simulink model "iiwa_model_tests"  (R2020b)
settings: Solver=VariableStepAuto  StartTime=0.0  StopTime=10.0  RelTol=1e-3
values from neighbouring files (symbols this model uses):
  q0 = zeros(7,1)    [setup.m]
undefined symbols (not defined in the file or in its folder): LWR, nofriction
libraries: roblocks x4
(part 2 of 2)

== matlab function iiwa_model_tests/inverse_dyn 1 ==
  data: q input; A output
function A = idm(q)

q1 = q(1);
q2 = q(2);
q3 = q(3);
q4 = q(4);
q5 = q(5);
q6 = q(6);
q7 = q(7);

radius = 0.05;

l1 = 0.1;
M1 = 2;

XX1 = 1/12 * M1 * l1 * l1;
XY1 = 0;
XZ1 = 0;
YY1 = 1/12 * M1 * l1 * l1;
YZ1 = 0;
ZZ1 = 1/2 * M1 * radius;
MX1 = 0;
MY1 = 0;
MZ1 = M1 * l1;

l2 = 0.1;
M2 = 2;

XX2 = 1/12 * M2 * l2 * l2;
XY2 = 0;
XZ2 = 0;
YY2 = 1/2 * M2 * radius;
YZ2 = 0;
ZZ2 = 1/12 * M2 * l2 * l2;
MX2 = 0;
MY2 = -M2 * l2;
MZ2 = 0;

l3 = 0.1;
M3 = 1.5;

XX3 = 1/12 * M3 * l3 * l3;
XY3 = 0;
XZ3 = 0;
YY3 = 1/12 * M3 * l3 * l3;
YZ3 = 0;
ZZ3 = 1/2 * M3 * radius;
MX3 = 0;
MY3 = 0;
MZ3 = M3 * l3;

l4 = 0.1;
M4 = 1.5;

XX4 = 1/12 * M4 * l4 * l4;
XY4 = 0;
XZ4 = 0;
YY4 = 1/2 * M4 * radius;
YZ4 = 0;
ZZ4 = 1/12 * M4 * l4 * l4;
MX4 = 0;
MY4 = M4 * 0.1;
MZ4 = 0;

l5 = 0.1;
M5 = 1.5;

XX5 = 1/12 * M5 * l5 * l5;
XY5 = 0;
XZ5 = 0;
YY5 = 1/12 * M5 * l5 * l5;
YZ5 = 0;
ZZ5 = 1/2 * M5 * radius;
MX5 = 0;
MY5 = 0;
MZ5 = M5 * l5;

l6 = 0.1;
M6 = 1;

XX6 = 1/12 * M6 * l6 * l6;
XY6 = 0;
XZ6 = 0;
YY6 = 1/12 * M6 * l6 * l6;
YZ6 = 0;
ZZ6 = 1/2 * M6 * radius;
MX6 = 0;
MY6 = -M6 * l6;
MZ6 = 0;

l7 = 0.05;
M7 = 0.1;

XX7 = 1/12 * M7 * l7 * l7;
XY7 = 0;
XZ7 = 0;
YY7 = 1/12 * M7 * l7 * l7;
YZ7 = 0;
ZZ7 = 1/2 * M7 * radius;
MX7 = 0;
MY7 = 0;
MZ7 = M7 * l7;


FX7 = 0;
FY7 = 0;
FZ7 = 0;
CX7 = 0;
CY7 = 0;
CZ7 = 0;
       
C1 = cos(q1);
S1 = sin(q1);
C2 = cos(q2);
S2 = sin(q2);
C3 = cos(q3);
S3 = sin(q3);
C4 = cos(q4);
S4 = sin(q4);
C5 = cos(q5);
S5 = sin(q5);
C6 = cos(q6);
S6 = sin(q6);
C7 = cos(q7);
S7 = sin(q7);
AS17 = C7*MX7 - MY7*S7;
AS37 = -C7*MY7 - MX7*S7;
AJ117 = C7*XX7;
AJ317 = -S7*XX7;
AJ127 = -S7*YY7;
AJ327 = -C7*YY7;
AJA117 = AJ117*C7 - AJ127*S7;
AJA317 = AJ317*C7 - AJ327*S7;
AJA137 = -AJ117*S7 - AJ127*C7;
AJA337 = -AJ317*S7 - AJ327*C7;
JP116 = AJA117 + XX6;
JP226 = YY6 + ZZ7;
JP336 = AJA337 + ZZ6;
MSP16 = AS17 + MX6;
MSP26 = MY6 + MZ7;
MSP36 = AS37 + MZ6;
MP6 = M6 + M7;
AS16 = C6*MSP16 - MSP26*S6;
AS36 = C6*MSP26 + MSP16*S6;
AJ116 = C6*JP116;
AJ316 = JP116*S6;
AJ126 = -JP226*S6;
AJ326 = C6*JP226;
AJ136 = AJA137*C6;
AJ336 = AJA137*S6;
AJA116 = AJ116*C6 - AJ126*S6;
AJA216 = -AJA317*C6;
AJA316 = AJ316*C6 - AJ326*S6;
AJA136 = AJ116*S6 + AJ126*C6;
AJA236 = -AJA317*S6;
AJA336 = AJ316*S6 + AJ326*C6;
JP115 = AJA116 + XX5;
JP225 = JP336 + YY5;
JP335 = AJA336 + ZZ5;
MSP15 = AS16 + MX5;
MSP25 = -MSP36 + MY5;
MSP35 = AS36 + MZ5;
MP5 = M5 + MP6;
AS15 = C5*MSP15 - MSP25*S5;
AS35 = C5*MSP25 + MSP15*S5;
AJ115 = -AJA216*S5 + C5*JP115;
AJ315 = AJA216*C5 + JP115*S5;
AJ125 = -AJ136*C5 - JP225*S5;
AJ325 = -AJ136*S5 + C5*JP225;
AJ135 = AJA136*C5 - AJA236*S5;
AJ335 = AJA136*S5 + AJA236*C5;
AJA115 = AJ115*C5 - AJ125*S5;
AJA215 = -AJ336*S5 - AJA316*C5;
AJA315 = AJ315*C5 - AJ325*S5;
AJA135 = AJ115*S5 + AJ125*C5;
AJA235 = AJ336*C5 - AJA316*S5;
AJA335 = AJ315*S5 + AJ325*C5;
PAS115 = -0.39*MSP35;
PAS125 = -0.39*AS15;
PAS325 = -0.39*AS35;
JP114 = AJA115 + 0.1521*MP5 - 2*PAS115 + XX4;
JP214 = AJA215 - PAS125;
JP124 = -AJ135 - PAS125;
JP224 = JP335 + YY4;
JP324 = -AJ335 - PAS325;
JP234 = AJA235 - PAS325;
JP334 = AJA335 + 0.1521*MP5 - 2*PAS115 + ZZ4;
MSP14 = AS15 + MX4;
MSP24 = -0.39*MP5 - MSP35 + MY4;
MSP34 = AS35 + MZ4;
MP4 = M4 + MP5;
AS14 = C4*MSP14 - MSP24*S4;
AS34 = -C4*MSP24 - MSP14*S4;
AJ114 = C4*JP114 - JP214*S4;
AJ314 = -C4*JP214 - JP114*S4;
AJ124 = C4*JP124 - JP224*S4;
AJ324 = -C4*JP224 - JP124*S4;
AJ134 = AJA135*C4 - JP234*S4;
AJ334 = -AJA135*S4 - C4*JP234;
AJA114 = AJ114*C4 - AJ124*S4;
AJA214 = AJA315*C4 - JP324*S4;
AJA314 = AJ314*C4 - AJ324*S4;
AJA134 = -AJ114*S4 - AJ124*C4;
AJA234 = -AJA315*S4 - C4*JP324;
AJA334 = -AJ314*S4 - AJ324*C4;
JP113 = AJA114 + XX3;
JP223 = JP334 + YY3;
JP333 = AJA334 + ZZ3;
MSP13 = AS14 + MX3;
MSP23 = MSP34 + MY3;
MSP33 = AS34 + MZ3;
MP3 = M3 + MP4;
AS13 = C3*MSP13 - MSP23*S3;
AS33 = -C3*MSP23 - MSP13*S3;
AJ113 = -AJA214*S3 + C3*JP113;
AJ313 = -AJA214*C3 - JP113*S3;
AJ123 = AJ134*C3 - JP223*S3;
AJ323 = -AJ134*S3 - C3*JP223;
AJ133 = AJA134*C3 - AJA234*S3;
AJ333 = -AJA134*S3 - AJA234*C3;
AJA113 = AJ113*C3 - AJ123*S3;
AJA213 = -AJ334*S3 + AJA314*C3;
AJA313 = AJ313*C3 - AJ323*S3;
AJA133 = -AJ113*S3 - AJ123*C3;
AJA233 = -AJ334*C3 - AJA314*S3;
AJA333 = -AJ313*S3 - AJ323*C3;
PAS113 = -0.4*MSP33;
PAS123 = 0.4*AS13;
PAS323 = 0.4*AS33;
JP112 = AJA113 + 0.16*MP3 - 2*PAS113 + XX2;
JP212 = AJA213 - PAS123;
JP122 = AJ133 - PAS123;
JP222 = JP333 + YY2;
JP322 = AJ333 - PAS323;
JP232 = AJA233 - PAS323;
JP332 = AJA333 + 0.16*MP3 - 2*PAS113 + ZZ2;
MSP12 = AS13 + MX2;
MSP22 = 0.4*MP3 + MSP33 + MY2;
MSP32 = AS33 + MZ2;
MP2 = M2 + MP3;
AS12 = C2*MSP12 - MSP22*S2;
AS32 = C2*MSP22 + MSP12*S2;
AJ112 = C2*JP112 - JP212*S2;
AJ312 = C2*JP212 + JP112*S2;
AJ122 = C2*JP122 - JP222*S2;
AJ322 = C2*JP222 + JP122*S2;
AJ132 = AJA133*C2 - JP232*S2;
AJ332 = AJA133*S2 + C2*JP232;
AJA112 = AJ112*C2 - AJ122*S2;
AJA212 = -AJA313*C2 + JP322*S2;
AJA312 = AJ312*C2 - AJ322*S2;
AJA132 = AJ112*S2 + AJ122*C2;
AJA232 = -AJA313*S2 - C2*JP322;
AJA332 = AJ312*S2 + AJ322*C2;
JP111 = AJA112 + XX1;
JP221 = JP332 + YY1;
JP331 = AJA332 + ZZ1;
MSP11 = AS12 + MX1;
MSP21 = -MSP32 + MY1;
MSP31 = AS32 + MZ1;
MP1 = M1 + MP2;
Nd12 = AJ133 - 0.4*C3*MSP13 + 0.4*MSP23*S3;
Nd32 = AJ333 + 0.4*C3*MSP23 + 0.4*MSP13*S3;
Ed11 = AS33*C2;
Ed31 = AS33*S2;
Nd11 = C2*Nd12 - JP333*S2;
Nd31 = C2*JP333 + Nd12*S2;
Ee12 = AS34*C3;
Ee32 = -AS34*S3;
Ne12 = AJ134*C3 - 0.4*AS34*S3 - JP334*S3;
Ne32 = -AJ134*S3 - 0.4*AS34*C3 - C3*JP334;
Ee11 = AS14*S2 + C2*Ee12;
Ee31 = -AS14*C2 + Ee12*S2;
Ne11 = -AJ334*S2 + C2*Ne12;
Ne31 = AJ334*C2 + Ne12*S2;
Nf14 = AJ135 - 0.39*C5*MSP15 + 0.39*MSP25*S5;
Nf34 = AJ335 - 0.39*C5*MSP25 - 0.39*MSP15*S5;
Ef13 = -AS35*C4;
Ef33 = AS35*S4;
Nf13 = C4*Nf14 + JP335*S4;
Nf33 = C4*JP335 - Nf14*S4;
Ef12 = -AS15*S3 + C3*Ef13;
Ef32 = -AS15*C3 - Ef13*S3;
Nf12 = -0.4*AS15*C3 + C3*Nf13 - 0.4*Ef13*S3 - Nf34*S3;
Nf32 = 0.4*AS15*S3 - 0.4*C3*Ef13 - C3*Nf34 - Nf13*S3;
Ef11 = C2*Ef12 - Ef33*S2;
Ef31 = C2*Ef33 + Ef12*S2;
Nf11 = C2*Nf12 - Nf33*S2;
Nf31 = C2*Nf33 + Nf12*S2;
Eg14 = -AS36*C5;
Eg34 = -AS36*S5;
Ng14 = AJ136*C5 + 0.39*AS36*S5 + JP336*S5;
Ng34 = AJ136*S5 - 0.39*AS36*C5 - C5*JP336;
Eg13 = AS16*S4 + C4*Eg14;
Eg33 = AS16*C4 - Eg14*S4;
Ng13 = AJ336*S4 + C4*Ng14;
Ng33 = AJ336*C4 - Ng14*S4;
Eg12 = C3*Eg13 - Eg34*S3;
Eg32 = -C3*Eg34 - Eg13*S3;
Ng12 = -0.4*C3*Eg34 + C3*Ng13 - 0.4*Eg13*S3 - Ng34*S3;
Ng32 = -0.4*C3*Eg13 - C3*Ng34 + 0.4*Eg34*S3 - Ng13*S3;
Eg11 = C2*Eg12 - Eg33*S2;
Eg31 = C2*Eg33 + Eg12*S2;
Ng11 = C2*Ng12 - Ng33*S2;
Ng31 = C2*Ng33 + Ng12*S2;
Eh15 = AS37*C6;
Eh35 = AS37*S6;
Nh15 = -S6*ZZ7;
Nh35 = C6*ZZ7;
Eh14 = -AS17*S5 + C5*Eh15;
Eh34 = AS17*C5 + Eh15*S5;
Nh14 = -0.39*AS17*C5 + C5*Nh15 - 0.39*Eh15*S5;
Nh34 = -0.39*AS17*S5 + 0.39*C5*Eh15 + Nh15*S5;
Eh13 = C4*Eh14 + Eh35*S4;
Eh33 = C4*Eh35 - Eh14*S4;
Nh13 = C4*Nh14 + Nh35*S4;
Nh33 = C4*Nh35 - Nh14*S4;
Eh12 = C3*Eh13 - Eh34*S3;
Eh32 = -C3*Eh34 - Eh13*S3;
Nh12 = -0.4*C3*Eh34 + C3*Nh13 - 0.4*Eh13*S3 - Nh34*S3;
Nh32 = -0.4*C3*Eh13 - C3*Nh34 + 0.4*Eh34*S3 - Nh13*S3;
Eh11 = C2*Eh12 - Eh33*S2;
Eh31 = C2*Eh33 + Eh12*S2;
Nh11 = C2*Nh12 - Nh33*S2;
Nh31 = C2*Nh33 + Nh12*S2;
A11 = JP331;
A21 = AJ332;
A31 = Nd31;
A41 = Ne31;
A51 = Nf31;
A61 = Ng31;
A71 = Nh31;
A22 = JP332;
A32 = Nd32;
A42 = Ne32;
A52 = Nf32;
A62 = Ng32;
A72 = Nh32;
A33 = JP333;
A43 = AJ334;
A53 = Nf33;
A63 = Ng33;
A73 = Nh33;
A44 = JP334;
A54 = Nf34;
A64 = Ng34;
A74 = Nh34;
A55 = JP335;
A65 = AJ336;
A75 = Nh35;
A66 = JP336;
A76 = 0;
A77 = ZZ7;

A1 = [
    A11 0   0   0   0   0   0;
    A21 A22 0   0   0   0   0;
    A31 A32 A33 0   0   0   0;
    A41 A42 A43 A44 0   0   0;
    A51 A52 A53 A54 A55 0   0;
    A61 A62 A63 A64 A65 A66 0;
    A71 A72 A73 A74 A75 A76 A77 
];

A = A1 + A1';
